simulink model "gm_ZynqBF_2tx_fpga"  (R2018b)
settings: Solver=FixedStepDiscrete  StartTime=0.0  StopTime=10.0  FixedStep=(1/420e3)/128  RelTol=1e-3
undefined symbols (not defined in the file or in its folder): a, b, c
libraries: hdlsllib x873, simulink x349
(part 1 of 40)
settings Model: Creator=jason  LastModifiedBy=jason
settings DataIOCC: SaveOutput=off  SaveTime=off
settings OptimizationCC: BlockReduction=off  ConditionallyExecuteInputs=off  DefaultParameterBehavior=Inlined
settings DebuggingCC: AlgebraicLoopMsg=error  InheritedTsInSrcMsg=none  SingleTaskRateTransMsg=error  ParameterPrecisionLossMsg=none  StrictBusMsg=ErrorOnBusTreatedAsVector
settings HardwareCC: ProdBitPerPointer=32  ProdBitPerSizeT=32  ProdBitPerPtrDiffT=32  ProdLargestAtomicFloat=None  ProdIntDivRoundTo=Undefined  ProdEndianess=Unspecified  ProdWordSize=32  ProdHWDeviceType=ASIC/FPGA->ASIC/FPGA  ProdEqTarget=off
settings SFSimCC: SimUseLocalCustomCode=off
settings RTWCC: RTWUseLocalCustomCode=off
settings CodeAppCC: StateflowObjectComments=on
settings GRTTargetCC: TargetLangStandard=C89/C90 (ANSI)

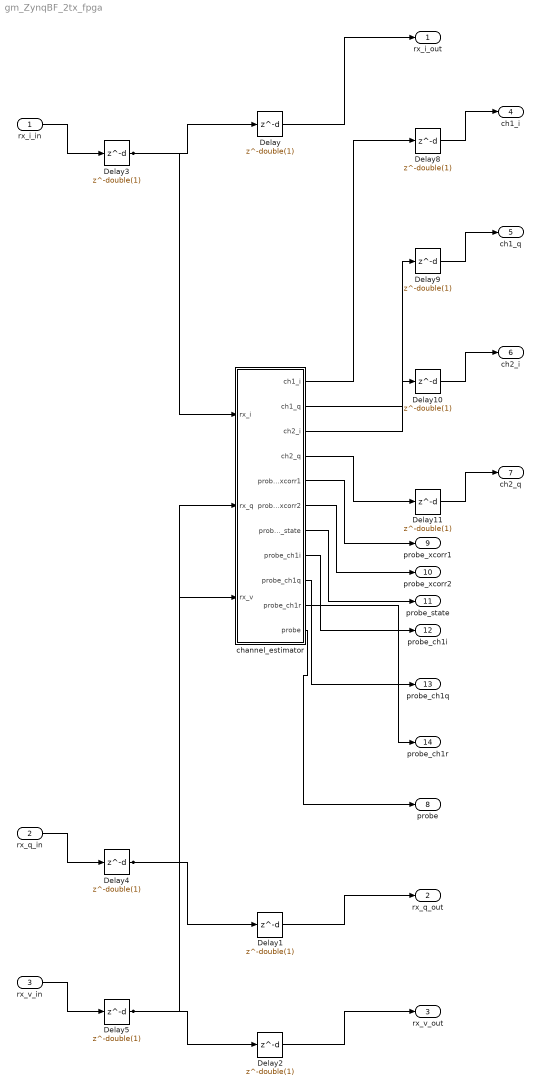
== system gm_ZynqBF_2tx_fpga ==
  rx_i_in : Inport  OutDataTypeStr=fixdt(1, 16, 15)  PortDimensions=1  SampleTime=2.38095238095238e-06
  rx_q_in : Inport  Port=2  OutDataTypeStr=fixdt(1, 16, 15)  PortDimensions=1  SampleTime=2.38095238095238e-06
  rx_v_in : Inport  Port=3  OutDataTypeStr=boolean  PortDimensions=1  SampleTime=2.38095238095238e-06
  Delay{,1..5} (6 alike) : Delay  DelayLength=double(1)  InitialCondition=0  InputProcessing=Inherited  SampleTime=2.38095238095238e-06
  Delay{8..11} (4 alike) : Delay  DelayLength=double(1)  InitialCondition=0  InputProcessing=Inherited  SampleTime=1.86011904761905e-08
  channel_estimator : Subsystem
  rx_i_out : Outport  OutDataTypeStr=fixdt(1,16,15)  SampleTime=1/420e3
  rx_q_out : Outport  Port=2  OutDataTypeStr=fixdt(1,16,15)  SampleTime=1/420e3
  rx_v_out : Outport  Port=3  OutDataTypeStr=boolean  SampleTime=1/420e3  LockScale=on
  ch1_i : Outport  Port=4  OutDataTypeStr=fixdt(1,16,15)
  ch1_q : Outport  Port=5  OutDataTypeStr=fixdt(1,16,15)
  ch2_i : Outport  Port=6  OutDataTypeStr=fixdt(1,16,15)
  ch2_q : Outport  Port=7  OutDataTypeStr=fixdt(1,16,15)
  probe : Outport  Port=8
  probe_xcorr1 : Outport  Port=9
  probe_xcorr2 : Outport  Port=10
  probe_state : Outport  Port=11
  probe_ch1i : Outport  Port=12
  probe_ch1q : Outport  Port=13
  probe_ch1r : Outport  Port=14
  wires:
  rx_i_in/1 -> Delay3/1
  rx_q_in/1 -> Delay4/1
  rx_v_in/1 -> Delay5/1
  Delay/1 -> rx_i_out/1
  Delay1/1 -> rx_q_out/1
  Delay10/1 -> ch2_i/1
  Delay11/1 -> ch2_q/1
  Delay2/1 -> rx_v_out/1
  Delay3/1 -> Delay/1, channel_estimator/1(rx_i)
  Delay4/1 -> Delay1/1, channel_estimator/2(rx_q)
  Delay5/1 -> Delay2/1, channel_estimator/3(rx_v)
  Delay8/1 -> ch1_i/1
  Delay9/1 -> ch1_q/1
  channel_estimator/1(ch1_i) -> Delay8/1
  channel_estimator/2(ch1_q) -> Delay9/1
  channel_estimator/3(ch2_i) -> Delay10/1
  channel_estimator/4(ch2_q) -> Delay11/1
  channel_estimator/5(probe_xcorr1) -> probe_xcorr1/1
  channel_estimator/6(probe_xcorr2) -> probe_xcorr2/1
  channel_estimator/7(probe_state) -> probe_state/1
  channel_estimator/8(probe_ch1i) -> probe_ch1i/1
  channel_estimator/9(probe_ch1q) -> probe_ch1q/1
  channel_estimator/10(probe_ch1r) -> probe_ch1r/1
  channel_estimator/11(probe) -> probe/1

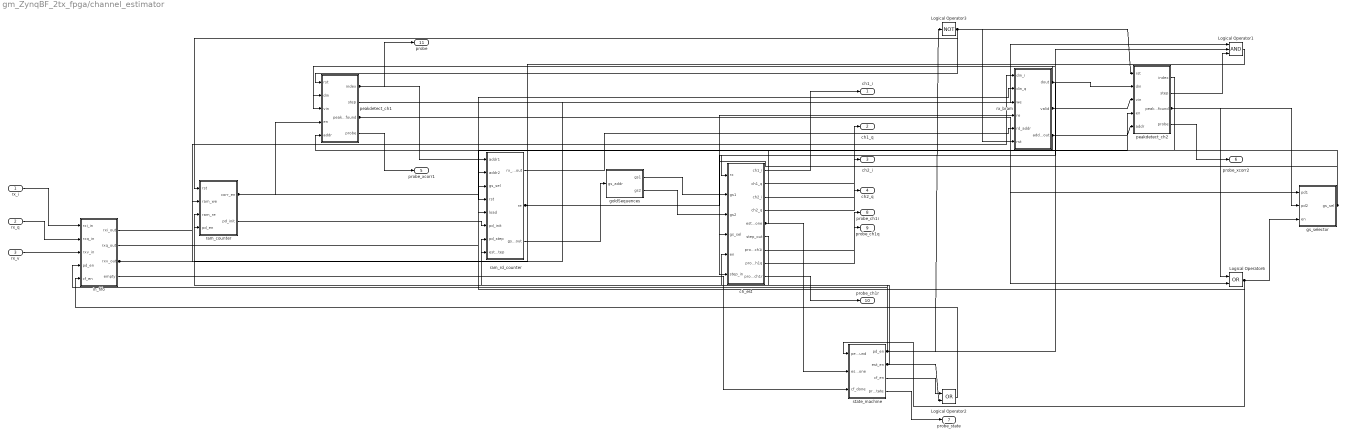
== system gm_ZynqBF_2tx_fpga/channel_estimator ==
  rx_i : Inport  OutDataTypeStr=fixdt(1, 16, 15)  PortDimensions=1  SampleTime=2.38095238095238e-06
  rx_q : Inport  Port=2  OutDataTypeStr=fixdt(1, 16, 15)  PortDimensions=1  SampleTime=2.38095238095238e-06
  rx_v : Inport  Port=3  OutDataTypeStr=boolean  PortDimensions=1  SampleTime=2.38095238095238e-06
  Logical Operator1 : Logic  Inputs=3  AllPortsSameDT=off  OutDataTypeStr=boolean  SampleTime=1.86011904761905e-08
  Logical Operator2 : Logic  Operator=OR  AllPortsSameDT=off  OutDataTypeStr=boolean  SampleTime=1.86011904761905e-08
  Logical Operator3 : Logic  Operator=NOT  Inputs=1  AllPortsSameDT=off  OutDataTypeStr=boolean  SampleTime=1.86011904761905e-08
  Logical Operator6 : Logic  Operator=OR  AllPortsSameDT=off  OutDataTypeStr=boolean  SampleTime=1.86011904761905e-08
  ch_est : Subsystem
  goldSequences : Subsystem
  gs_selector : Subsystem
  in_fifo : Subsystem
  peakdetect_ch1 : Subsystem
  peakdetect_ch2 : Subsystem
  ram_counter : Subsystem
  ram_rd_counter : Subsystem
  rx_bram : Subsystem
  state_machine : Subsystem
  ch1_i : Outport
  ch1_q : Outport  Port=2
  ch2_i : Outport  Port=3
  ch2_q : Outport  Port=4
  probe_xcorr1 : Outport  Port=5
  probe_xcorr2 : Outport  Port=6
  probe_state : Outport  Port=7
  probe_ch1i : Outport  Port=8
  probe_ch1q : Outport  Port=9
  probe_ch1r : Outport  Port=10
  probe : Outport  Port=11
  wires:
  rx_i/1 -> in_fifo/1(rxi_in)
  rx_q/1 -> in_fifo/2(rxq_in)
  rx_v/1 -> in_fifo/3(rxv_in)
  ch_est/1(ch1_i) -> ch1_i/1
  ch_est/2(ch1_q) -> ch1_q/1
  ch_est/3(ch2_i) -> ch2_i/1
  ch_est/4(ch2_q) -> ch2_q/1
  ch_est/7(probe_ch1i) -> probe_ch1i/1
  ch_est/8(probe_ch1q) -> probe_ch1q/1
  ch_est/9(probe_ch1r) -> probe_ch1r/1
  peakdetect_ch1/1(index) -> probe/1, ram_rd_counter/1(addr1)
  peakdetect_ch1/4(probe) -> probe_xcorr1/1
  peakdetect_ch2/4(probe) -> probe_xcorr2/1
  state_machine/4(probe_state) -> probe_state/1
  goldSequences/1(gs1) -> ch_est/2(gs1)
  goldSequences/2(gs2) -> ch_est/3(gs2)
  Logical Operator2/1 -> in_fifo/5(cf_en)
  Logical Operator1/1 -> ram_rd_counter/7(pd_step)
  Logical Operator6/1 -> state_machine/1(peak_found), ram_rd_counter/5(load), gs_selector/3(en)
  gs_selector/1(gs_sel) -> ch_est/4(gs_sel), ram_rd_counter/3(gs_sel)
  peakdetect_ch1/2(step) -> Logical Operator1/1
  peakdetect_ch1/3(peak_found) -> Logical Operator6/2, gs_selector/1(pd1)
  ram_rd_counter/1(rx_addr_out) -> rx_bram/5(rd_addr)
  ram_rd_counter/2(re) -> ram_counter/3(ram_re), rx_bram/4(re)
  ram_rd_counter/3(gs_addr_out) -> goldSequences/1(gs_addr)
  ram_counter/1(corr_en) -> peakdetect_ch2/4(en), peakdetect_ch1/4(en)
  ram_counter/2(pd_init) -> ram_rd_counter/6(pd_init)
  Logical Operator3/1 -> ram_counter/1(rst), peakdetect_ch2/1(rst), peakdetect_ch1/1(rst), rx_bram/6(rst)
  peakdetect_ch2/1(index) -> ram_rd_counter/2(addr2)
  peakdetect_ch2/2(step) -> Logical Operator1/3
  peakdetect_ch2/3(peak_found) -> Logical Operator6/1, gs_selector/2(pd2)
  state_machine/1(pd_en) -> Logical Operator3/1, Logical Operator1/2, in_fifo/4(pd_en), ram_counter/4(pd_en)
  state_machine/2(est_en) -> Logical Operator2/2, ch_est/5(en)
  state_machine/3(cf_en) -> Logical Operator2/1
  in_fifo/1(rxi_out) -> rx_bram/1(din_i)
  in_fifo/2(rxq_out) -> rx_bram/2(din_q)
  in_fifo/3(rxv_out) -> ram_counter/2(ram_we), rx_bram/3(we)
  in_fifo/4(empty) -> state_machine/3(cf_done)
  rx_bram/1(dout) -> ch_est/1(rx), peakdetect_ch2/2(din), peakdetect_ch1/2(din)
  rx_bram/2(valid) -> peakdetect_ch2/3(vin), ch_est/6(step_in), peakdetect_ch1/3(vin)
  rx_bram/3(addr_out) -> peakdetect_ch2/5(addr), peakdetect_ch1/5(addr)
  ch_est/5(est_done) -> ram_rd_counter/4(rst), state_machine/2(est_done)
  ch_est/6(step_out) -> ram_rd_counter/8(est_step)

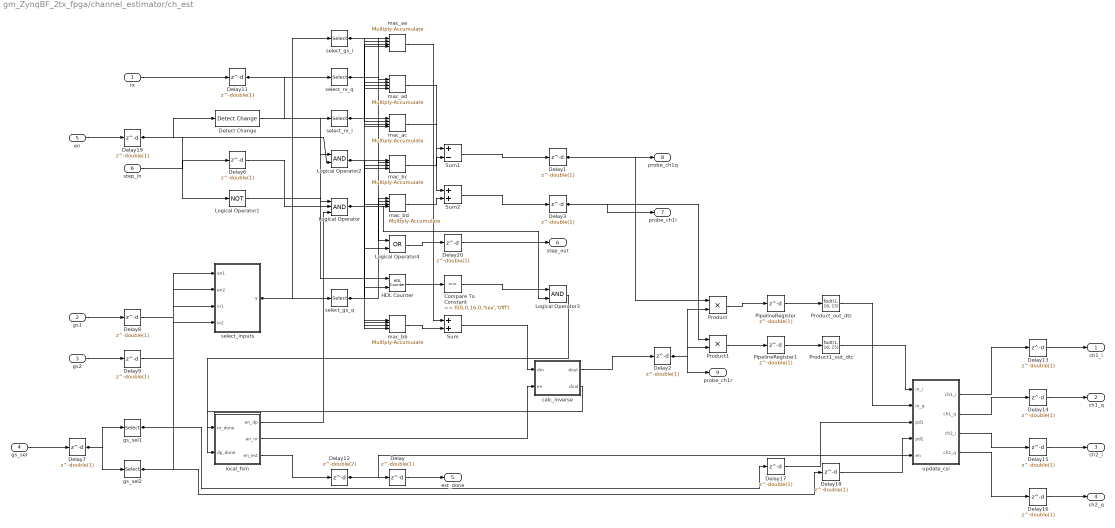
== system gm_ZynqBF_2tx_fpga/channel_estimator/ch_est ==
  rx : Inport  OutDataTypeStr=fixdt(1, 16, 15)  PortDimensions=[2]  SampleTime=1.86011904761905e-08
  gs1 : Inport  Port=2  OutDataTypeStr=fixdt(1, 16, 15)  PortDimensions=[2]  SampleTime=1.86011904761905e-08
  gs2 : Inport  Port=3  OutDataTypeStr=fixdt(1, 16, 15)  PortDimensions=[2]  SampleTime=1.86011904761905e-08
  gs_sel : Inport  Port=4  OutDataTypeStr=boolean  PortDimensions=[2]  SampleTime=1.86011904761905e-08
  en : Inport  Port=5  OutDataTypeStr=boolean  PortDimensions=1  SampleTime=1.86011904761905e-08
  step_in : Inport  Port=6  OutDataTypeStr=boolean  PortDimensions=1  SampleTime=1.86011904761905e-08
  Compare To Constant : simulink/Logic and Bit Operations/Compare To Constant  relop===  const=fi(0,0,16,0,'hex','0fff')  OutDataTypeStr=boolean
  Delay{,1..3,6..9,11,13..20} (17 alike) : Delay  DelayLength=double(1)  InitialCondition=0  InputProcessing=Inherited  SampleTime=1.86011904761905e-08
  Delay12 : Delay  DelayLength=double(2)  InitialCondition=0  InputProcessing=Inherited  SampleTime=1.86011904761905e-08
  Detect Change : simulink/Logic and Bit Operations/Detect Change  vinit=0  OutDataTypeStr=boolean
  HDL Counter : hdlsllib/Sources/HDL Counter  CountType=Count limited  CountInit=double(0)  CountStep=double(1)  CountMax=double(4095)  CountFromType=Initial value  CountFrom=double(0)  CountResetPort=on  CountLoadPort=off  CountEnbPort=on  CountDirPort=off  CountDataType=Unsigned  CountWordLen=16  CountFracLen=0  CountSampTime=1.86011904761905e-08
      settings: SourceProductBaseCode=HD
  Logical Operator : Logic  Inputs=3  AllPortsSameDT=off  OutDataTypeStr=boolean  SampleTime=1.86011904761905e-08
  Logical Operator1 : Logic  Operator=NOT  Inputs=1  AllPortsSameDT=off  OutDataTypeStr=boolean  SampleTime=1.86011904761905e-08
  Logical Operator2 : Logic  AllPortsSameDT=off  OutDataTypeStr=boolean  SampleTime=1.86011904761905e-08
  Logical Operator3 : Logic  AllPortsSameDT=off  OutDataTypeStr=boolean  SampleTime=1.86011904761905e-08
  Logical Operator4 : Logic  Operator=OR  AllPortsSameDT=off  OutDataTypeStr=boolean  SampleTime=1.86011904761905e-08
  PipelineRegister : Delay  DelayLength=double(1)  InitialCondition=0  InputProcessing=Inherited  SampleTime=1.86011904761905e-08
  PipelineRegister1 : Delay  DelayLength=double(1)  InitialCondition=0  InputProcessing=Inherited  SampleTime=1.86011904761905e-08
  Product : Product  Inputs=**  OutDataTypeStr=fixdt(1, 64, 30)  SampleTime=1.86011904761905e-08
  Product1 : Product  Inputs=**  OutDataTypeStr=fixdt(1, 64, 30)  SampleTime=1.86011904761905e-08
  Product1_out_dtc : DataTypeConversion  OutDataTypeStr=fixdt(1, 16, 15)  SampleTime=1.86011904761905e-08
  Product_out_dtc : DataTypeConversion  OutDataTypeStr=fixdt(1, 16, 15)  SampleTime=1.86011904761905e-08
  Sum : Sum  AccumDataTypeStr=fixdt(1, 33, 16)  OutDataTypeStr=fixdt(1, 32, 16)  SampleTime=1.86011904761905e-08
  Sum1 : Sum  Inputs=+-  AccumDataTypeStr=fixdt(1, 33, 16)  OutDataTypeStr=fixdt(1, 32, 16)  SampleTime=1.86011904761905e-08
  Sum2 : Sum  AccumDataTypeStr=fixdt(1, 33, 16)  OutDataTypeStr=fixdt(1, 32, 16)  SampleTime=1.86011904761905e-08
  calc_inverse : Subsystem
  gs_sel1 : Selector  IndexMode=Zero-based  SampleTime=1.86011904761905e-08  IndexOptions=Index vector (dialog)  Indices=double(0)  OutputSizes=double(1)
  gs_sel2 : Selector  IndexMode=Zero-based  SampleTime=1.86011904761905e-08  IndexOptions=Index vector (dialog)  Indices=double(1)  OutputSizes=double(1)
  local_fsm : Subsystem
  mac_aa : hdlsllib/HDL Operations/Multiply-Accumulate  opMode=Streaming - using Start and End ports  initValueSetting=Dialog  initValue=0  initValueSetting2=Dialog  initValue2=0  initValueSetting3=Dialog  initValue3=0  num_samples=2  RndMeth2=Floor  RndMeth3=Floor  datatype2=fixdt(1, 32, 16)  datatype3=Inherit: Inherit via back propagation  validOut=off  endInandOut=off  startOut=off  countOut=on  dim=-1  DoSatur=off  parallel=off
      settings: SourceProductName=HDL Coder  SourceProductBaseCode=HD
  mac_ac : hdlsllib/HDL Operations/Multiply-Accumulate  opMode=Streaming - using Start and End ports  initValueSetting=Dialog  initValue=0  initValueSetting2=Dialog  initValue2=0  initValueSetting3=Dialog  initValue3=0  num_samples=2  RndMeth2=Floor  RndMeth3=Floor  datatype2=fixdt(1, 32, 16)  datatype3=Inherit: Inherit via back propagation  validOut=off  endInandOut=off  startOut=off  countOut=on  dim=-1  DoSatur=off  parallel=off
      settings: SourceProductName=HDL Coder  SourceProductBaseCode=HD
  mac_ad : hdlsllib/HDL Operations/Multiply-Accumulate  opMode=Streaming - using Start and End ports  initValueSetting=Dialog  initValue=0  initValueSetting2=Dialog  initValue2=0  initValueSetting3=Dialog  initValue3=0  num_samples=2  RndMeth2=Floor  RndMeth3=Floor  datatype2=fixdt(1, 32, 16)  datatype3=Inherit: Inherit via back propagation  validOut=off  endInandOut=off  startOut=off  countOut=on  dim=-1  DoSatur=off  parallel=off
      settings: SourceProductName=HDL Coder  SourceProductBaseCode=HD
  mac_bb : hdlsllib/HDL Operations/Multiply-Accumulate  opMode=Streaming - using Start and End ports  initValueSetting=Dialog  initValue=0  initValueSetting2=Dialog  initValue2=0  initValueSetting3=Dialog  initValue3=0  num_samples=2  RndMeth2=Floor  RndMeth3=Floor  datatype2=fixdt(1, 32, 16)  datatype3=Inherit: Inherit via back propagation  validOut=off  endInandOut=off  startOut=off  countOut=on  dim=-1  DoSatur=off  parallel=off
      settings: SourceProductName=HDL Coder  SourceProductBaseCode=HD
  mac_bc : hdlsllib/HDL Operations/Multiply-Accumulate  opMode=Streaming - using Start and End ports  initValueSetting=Dialog  initValue=0  initValueSetting2=Dialog  initValue2=0  initValueSetting3=Dialog  initValue3=0  num_samples=2  RndMeth2=Floor  RndMeth3=Floor  datatype2=fixdt(1, 32, 16)  datatype3=Inherit: Inherit via back propagation  validOut=off  endInandOut=off  startOut=off  countOut=on  dim=-1  DoSatur=off  parallel=off
      settings: SourceProductName=HDL Coder  SourceProductBaseCode=HD
  mac_bd : hdlsllib/HDL Operations/Multiply-Accumulate  opMode=Streaming - using Start and End ports  initValueSetting=Dialog  initValue=0  initValueSetting2=Dialog  initValue2=0  initValueSetting3=Dialog  initValue3=0  num_samples=2  RndMeth2=Floor  RndMeth3=Floor  datatype2=fixdt(1, 32, 16)  datatype3=Inherit: Inherit via back propagation  validOut=off  endInandOut=off  startOut=off  countOut=on  dim=-1  DoSatur=off  parallel=off
      settings: SourceProductName=HDL Coder  SourceProductBaseCode=HD
  select_gs_i : Selector  IndexMode=Zero-based  SampleTime=1.86011904761905e-08  IndexOptions=Index vector (dialog)  Indices=double(0)  OutputSizes=double(1)
  select_gs_q : Selector  IndexMode=Zero-based  SampleTime=1.86011904761905e-08  IndexOptions=Index vector (dialog)  Indices=double(1)  OutputSizes=double(1)
  select_inputs : Subsystem
  select_rx_i : Selector  IndexMode=Zero-based  SampleTime=1.86011904761905e-08  IndexOptions=Index vector (dialog)  Indices=double(0)  OutputSizes=double(1)
  select_rx_q : Selector  IndexMode=Zero-based  SampleTime=1.86011904761905e-08  IndexOptions=Index vector (dialog)  Indices=double(1)  OutputSizes=double(1)
  update_csi : Subsystem
  ch1_i : Outport
  ch1_q : Outport  Port=2
  ch2_i : Outport  Port=3
  ch2_q : Outport  Port=4
  est_done : Outport  Port=5
  step_out : Outport  Port=6
  probe_ch1i : Outport  Port=7
  probe_ch1q : Outport  Port=8
  probe_ch1r : Outport  Port=9
  wires:
  rx/1 -> Delay11/1
  gs1/1 -> Delay8/1
  gs2/1 -> Delay9/1
  gs_sel/1 -> Delay7/1
  en/1 -> Delay19/1
  step_in/1 -> Delay6/1
  Compare To Constant/1 -> Logical Operator3/1
  Delay/1 -> est_done/1
  Delay1/1 -> Product/1, probe_ch1q/1
  Delay11/1 -> select_rx_q/1, select_rx_i/1
  Delay12/1 -> Delay/1, update_csi/5(en)
  Delay13/1 -> ch1_i/1
  Delay14/1 -> ch1_q/1
  Delay15/1 -> ch2_i/1
  Delay16/1 -> ch2_q/1
  Delay17/1 -> update_csi/3(pd1)
  Delay18/1 -> update_csi/4(pd2)
  Delay19/1 -> Logical Operator2/2, Logical Operator1/1, Logical Operator/1, Detect Change/1
  Delay2/1 -> Product1/2, Product/2, probe_ch1r/1
  Delay20/1 -> step_out/1
  Delay3/1 -> Product1/1, probe_ch1i/1
  Delay6/1 -> Logical Operator/2
  Delay7/1 -> gs_sel2/1, gs_sel1/1
  Delay8/1 -> select_inputs/3(in1)
  Delay9/1 -> select_inputs/4(in2)
  Detect Change/1 -> Logical Operator2/1
  HDL Counter/1 -> Compare To Constant/1
  Logical Operator/1 -> Logical Operator4/2, Logical Operator3/2, mac_bd/4, mac_bc/4, mac_bb/4, mac_ad/4, mac_ac/4, mac_aa/4, HDL Counter/2
  Logical Operator1/1 -> HDL Counter/1
  Logical Operator2/1 -> Logical Operator4/1, mac_bd/3, mac_bc/3, mac_bb/3, mac_ad/3, mac_ac/3, mac_aa/3
  Logical Operator3/1 -> local_fsm/2(dp_done)
  Logical Operator4/1 -> Delay20/1
  Product_out_dtc/1 -> update_csi/2(in_q)
  Product1_out_dtc/1 -> update_csi/1(in_i)
  Sum/1 -> calc_inverse/1(din)
  Sum1/1 -> Delay1/1
  Sum2/1 -> Delay3/1
  calc_inverse/1(dout) -> Delay2/1
  calc_inverse/2(dval) -> local_fsm/1(nr_done)
  gs_sel1/1 -> Delay17/1, select_inputs/1(en1)
  gs_sel2/1 -> Delay18/1, select_inputs/2(en2)
  local_fsm/1(en_dp) -> Logical Operator/3
  local_fsm/2(en_nr) -> calc_inverse/2(en)
  local_fsm/3(en_est) -> Delay12/1
  mac_aa/1 -> Sum/1
  mac_ac/1 -> Sum2/1
  mac_ad/1 -> Sum1/1
  mac_bb/1 -> Sum/2
  mac_bc/1 -> Sum1/2
  mac_bd/1 -> Sum2/2
  select_gs_i/1 -> mac_ad/1, mac_ac/1, mac_aa/2, mac_aa/1
  select_gs_q/1 -> mac_bd/1, mac_bc/1, mac_bb/2, mac_bb/1
  select_inputs/1(y) -> select_gs_q/1, select_gs_i/1
  select_rx_i/1 -> mac_bc/2, mac_ac/2
  select_rx_q/1 -> mac_bd/2, mac_ad/2
  update_csi/1(ch1_i) -> Delay13/1
  update_csi/2(ch1_q) -> Delay14/1
  update_csi/3(ch2_i) -> Delay15/1
  update_csi/4(ch2_q) -> Delay16/1
  PipelineRegister/1 -> Product_out_dtc/1
  PipelineRegister1/1 -> Product1_out_dtc/1
  Product/1 -> PipelineRegister/1
  Product1/1 -> PipelineRegister1/1
